simulink model "Lab03b"  (Simulink 7.4)
settings: Solver=ode23tb  StartTime=0.0  StopTime=0.5  MaxStep=100e-6  RelTol=1e-3
libraries: powerlib x8, powerlib_extras x1
settings Model: Creator=msse8  LastModifiedBy=msse8

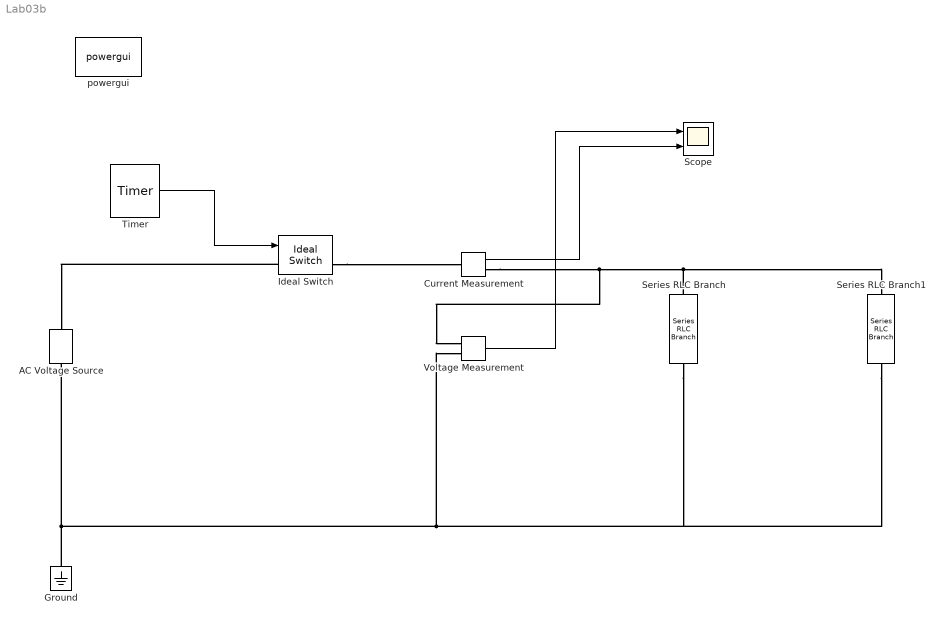
== system Lab03b ==
  AC Voltage Source : powerlib/Electrical Sources/AC Voltage Source  DialogController=POWERSYS.PowerSysDialog  SystemSampleTime=-1  Amplitude=230  Phase=0  Frequency=50  SampleTime=0  Measurements=None
  Current Measurement : powerlib/Measurements/Current Measurement  DialogController=POWERSYS.PowerSysDialog  SystemSampleTime=-1  PhasorSimulation=off  OutputType=Complex  PSBequivalent=0
  Ground : powerlib/Elements/Ground  DialogController=POWERSYS.PowerSysDialog  PhysicalDomain=powersysdomain  SubClassName=unknown  LeftPortType=p1  RightPortType=p1  LConnTagsString=a
  Ideal Switch : powerlib/Power Electronics/Ideal Switch  DialogController=POWERSYS.PowerSysDialog  SystemSampleTime=-1  Ron=0.001  Lon=0  IC=0  Rs=1e5  Cs=inf  Measurements=on
  Scope : Scope  NumInputPorts=2
      settings: YMin=-5~-5  YMax=5~5
  Series RLC Branch : powerlib/Elements/Series RLC Branch  DialogController=POWERSYS.PowerSysDialog  PhysicalDomain=powersysdomain  SubClassName=unknown  LeftPortType=p1  RightPortType=p1  LConnTagsString=__new0  RConnTagsString=__new0  BranchType=RL  Resistance=10  Inductance=0.1e-3  SetiL0=off  InitialCurrent=0  Capacitance=1e-6  Setx0=off  InitialVoltage=0  Measurements=None
  Series RLC Branch1 : powerlib/Elements/Series RLC Branch  DialogController=POWERSYS.PowerSysDialog  PhysicalDomain=powersysdomain  SubClassName=unknown  LeftPortType=p1  RightPortType=p1  LConnTagsString=__new0  RConnTagsString=__new0  BranchType=C  Resistance=1  Inductance=1e-3  SetiL0=off  InitialCurrent=0  Capacitance=10e-6  Setx0=off  InitialVoltage=0  Measurements=None
  Timer : powerlib_extras/Control  Blocks/Timer  DialogController=POWERSYS.PowerSysDialog  SystemSampleTime=-1  t="[ 0  5/50 ]"  e="[1  0]"
  Voltage Measurement : powerlib/Measurements/Voltage Measurement  DialogController=POWERSYS.PowerSysDialog  SystemSampleTime=-1  PhasorSimulation=off  OutputType=Complex  PSBequivalent=0
  powergui : powerlib/powergui  Priority=1  SystemSampleTime=-1  SimulationMode=Continuous  SampleTime=50e-6  frequency=60  SPID=off  DisableSnubberDevices=off  DisableRonSwitches=off  DisableVfSwitches=off  SwTol=0  Interpol=off  frequencyindice=50  echomessages=off  HookPort=off  DisplayEquations=off  FunctionMessages=off  EnableUseOfTLC=off  x0status=blocks  RestoreLinks=warning  Frange=[0:2:500]  Ylog=off  Xlog=on  ShowGrid=off  save=off  variable=ZData  ZoomFFT=on  StartTime=0.0  cycles=1  DisplayStyle=1  fundamental=60  FreqAxis=off  MaxFrequency=1000  frequencyindicesteady=1  RmsSteady=1  display=off  Ts=0  methode=off
  wires:
  Timer/1 -> Ideal Switch/1
  Current Measurement/1 -> Scope/2
  Voltage Measurement/1 -> Scope/1
  connections:
  Series RLC Branch1/RConn1 -- Series RLC Branch/RConn1 -- Ground/LConn1 -- AC Voltage Source/LConn1 -- Voltage Measurement/LConn2
  Ideal Switch/LConn1 -- AC Voltage Source/RConn1
  Current Measurement/RConn1 -- Series RLC Branch/LConn1 -- Series RLC Branch1/LConn1 -- Voltage Measurement/LConn1
  Ideal Switch/RConn1 -- Current Measurement/LConn1
